simulink model "chemostat"  (R2024b)
settings: Solver=VariableStepAuto  StartTime=0.0  StopTime=100  RelTol=1e-3
settings Model: Creator=Botló  LastModifiedBy=Botló

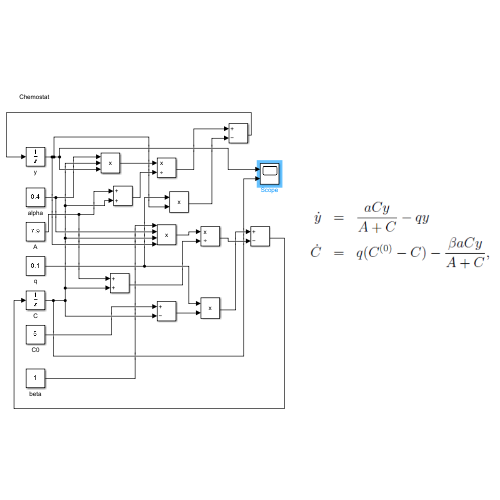
[thumbnail: Simulink's stored preview of the top-level diagram]
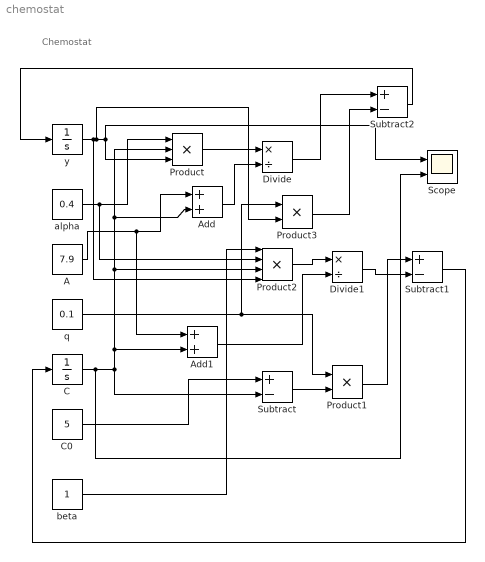
== system chemostat ==
  note: Chemostat
  A : Constant  Value=7.9
  Add : Sum
  Add1 : Sum
  C : Integrator  InitialCondition=10
  C0 : Constant  Value=5
  Divide : Product  Inputs=*/
  Divide1 : Product  Inputs=*/
  Product : Product  Inputs=3
  Product1 : Product
  Product2 : Product  Inputs=4
  Product3 : Product
  Scope : Scope  NumInputPorts=2
  Subtract : Sum  Inputs=+-
  Subtract1 : Sum  Inputs=+-
  Subtract2 : Sum  Inputs=+-
  alpha : Constant  Value=0.4
  beta : Constant
  q : Constant  Value=0.1
  y : Integrator  InitialCondition=5
  wires:
  alpha/1 -> Product2/2, Product/1
  y/1 -> Product3/2, Scope/1, Product/3, Product2/4
  C/1 -> Scope/2, Subtract/2, Add1/2, Product/2, Add/2, Product2/3
  A/1 -> Add1/1, Add/1
  Product/1 -> Divide/1
  Add/1 -> Divide/2
  Divide/1 -> Subtract2/1
  Product3/1 -> Subtract2/2
  q/1 -> Product1/1, Product3/1
  Subtract2/1 -> y/1
  C0/1 -> Subtract/1
  Subtract/1 -> Product1/2
  Product1/1 -> Subtract1/1
  beta/1 -> Product2/1
  Product2/1 -> Divide1/1
  Add1/1 -> Divide1/2
  Divide1/1 -> Subtract1/2
  Subtract1/1 -> C/1
